simulink model "Variant_System"  (R2025b)
settings: Solver=FixedStepDiscrete  StartTime=0.0  StopTime=10.0  FixedStep=0.01  RelTol=1e-3
settings Model: Creator=soura  LastModifiedBy=soura

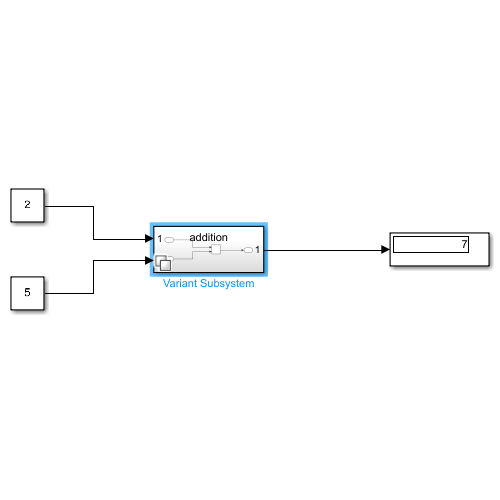
[thumbnail: Simulink's stored preview of the top-level diagram]
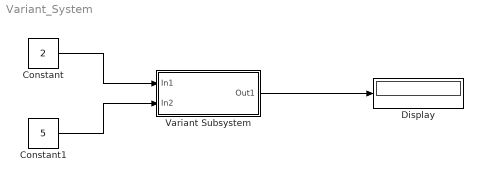
== system Variant_System ==
  Constant : Constant  Value=2
  Constant1 : Constant  Value=5
  Display : Display
  Variant Subsystem : Subsystem  InitFcn=var=Simulink.Variant('Calc==0')  Variant=on
  wires:
  Constant/1 -> Variant Subsystem/1(In1)
  Constant1/1 -> Variant Subsystem/2(In2)
  Variant Subsystem/1(Out1) -> Display/1

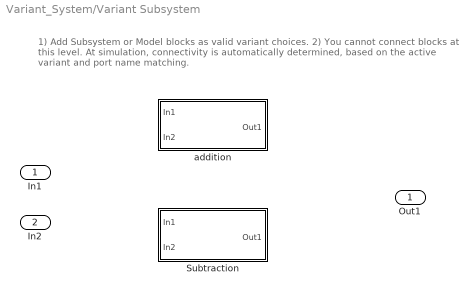
== system Variant_System/Variant Subsystem ==
  note: 1) Add Subsystem or Model blocks as valid variant choices.
      | 2) You cannot connect blocks at this level. At simulation, connectivity is automatically
      | determined, based on the active variant and port name matching.
  In1 : Inport
  In2 : Inport  Port=2
  Subtraction : Subsystem  VariantControl=Calc==1
  addition : Subsystem  VariantControl=Calc==0
  Out1 : Outport

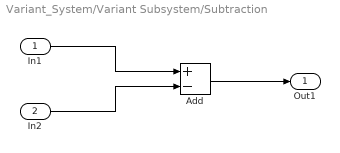
== system Variant_System/Variant Subsystem/Subtraction ==
  In1 : Inport
  In2 : Inport  Port=2
  Add : Sum  Inputs=+-
  Out1 : Outport
  wires:
  In1/1 -> Add/1
  Add/1 -> Out1/1
  In2/1 -> Add/2

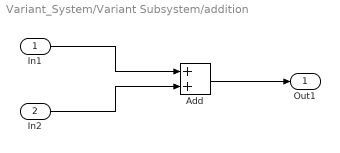
== system Variant_System/Variant Subsystem/addition ==
  In1 : Inport
  In2 : Inport  Port=2
  Add : Sum
  Out1 : Outport
  wires:
  Add/1 -> Out1/1
  In1/1 -> Add/1
  In2/1 -> Add/2
